simulink model "SMC_GRNN_Controller"  (R2019b)
settings: Solver=FixedStepAuto  StartTime=0.0  StopTime=60  FixedStep=1e-2  RelTol=1e-3
settings Model: Creator=Ivan Lopez  LastModifiedBy=Ivan Lopez

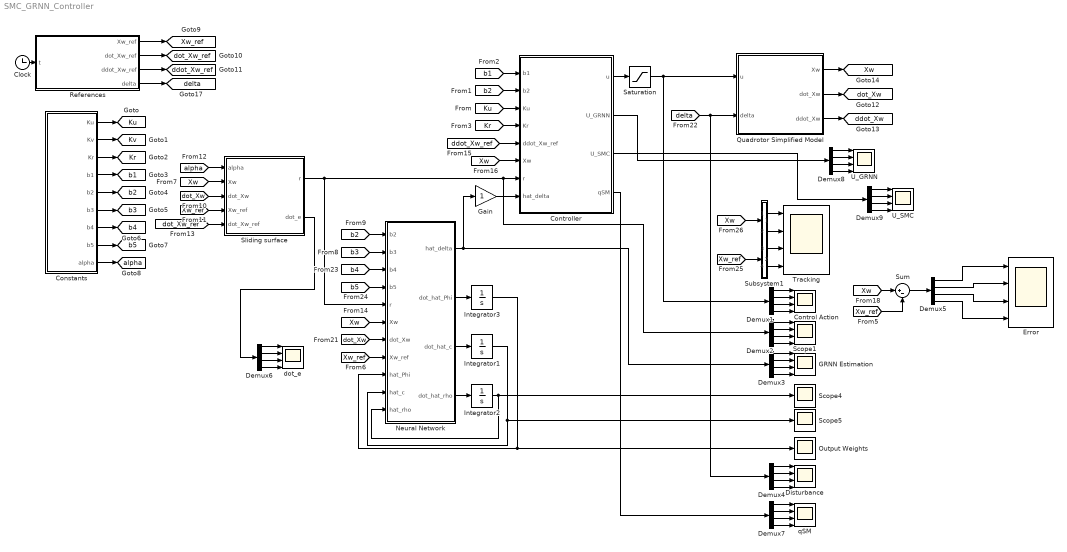
== system SMC_GRNN_Controller ==
  Clock : Clock
  Constants : MATLAB Function  TreatAsAtomicUnit=on
  Control Action : Scope  NumInputPorts=4
  Controller : MATLAB Function  TreatAsAtomicUnit=on
  Demux{1..9} (9 alike) : Demux
  Disturbance : Scope  NumInputPorts=4
  Error : Scope  NumInputPorts=4
  GRNN Estimation : Scope  NumInputPorts=4
  Gain : Gain
  Integrator1 : Integrator  InitialCondition=|
      | [0.6294
      |     0.8116
      |    -0.7460
      |     0.8268
      |     0.2647
      |    -0.8049
      |    -0.4430
      |     0.0938
      |     0.9150
      |     0.9298
      |    -0.6848
      |     0.9412
      |     0.9143
      |    -0.0292
      |     0.6006
      |    -0.7162
      |    -0.1565
      |     0.8315
      |     0.5844
      |     0.9190
      |     0.3115
      |    -0.9286
      |     0.6983
      |     0.8680
      |     0.3575
      |     0.5155
      |     0.4863
      |    -0.2155
      |     0.3110
      |    -0.6576
      |     0.4121
      |    -0.9363
      |    -0.4462
      |    -0.9077
      |    -0.8057
      |     0.6469
      |     0.3897
      |    -0.3658
      |     0.9004
      |    -0.9311
      |    -0.1225
      |    -0.2369
      |     0.5310
      |     0.5904
      |    -0.6263
      |    -0.0205
      |    -0.1088
      |     0.2926
      |     0.4187
      |     0.5094
      |    -0.4479
      |     0.3594
      |     0.3102
      |    -0.6748
      |    -0.7620
      |    -0.0033
      |     0.9195
      |    -0.3192
      |     0.1705
      |    -0.5524
      |     0.5025
      |    -0.4898
      |     0.0119
      |     0.3982
      |     0.7818
      |     0.9186
      |     0.0944
      |    -0.7228
      |    -0.7014
      |    -0.4850
      |     0.6814
      |    -0.4914
      |     0.6286
      |    -0.5130
      |     0.8585
      |    -0.3000
      |    -0.6068
      |    -0.4978
      |     0.2321
      |    -0.0534
      |    -0.2967
      |     0.6617
      |     0.1705
      |     0.0994
      |     0.8344
      |    -0.4283
      |     0.5144
      |     0.5075
      |    -0.2391
      |     0.1356
      |    -0.8483
      |    -0.8921
      |     0.0616
      |     0.5583
      |     0.8680
      |    -0.7402
      |     0.1376
      |    -0.0612
      |    -0.9762
      |    -0.3258
      |    -0.6756
      |     0.5886
      |    -0.3776
      |     0.0571
      |    -0.6687
      |     0.2040
      |    -0.4741
      |     0.3082
      |     0.3784
      |     0.4963
      |    -0.0989
      |    -0.8324
      |    -0.5420
      |     0.8267
      |    -0.6952
      |     0.6516
      |     0.0767
      |     0.9923
      |    -0.8436
      |    -0.1146
      |    -0.7867
      |     0.9238
      |    -0.9907
      |     0.5498
      |     0.6346
      |     0.7374
      |    -0.8311
      |    -0.2004
      |    -0.4803
      |     0.6001]'
  Integrator2 : Integrator  InitialCondition=ones(10,1)
  Integrator3 : Integrator  InitialCondition=|
      | [0.6628   -0.9690   -0.8946    0.3327;
      |     0.6067    0.9681    0.4757    0.0783;
      |    -0.8791   -0.6657   -0.4618    0.3962;
      |    -0.2015   -0.7876   -0.1543    0.3331;
      |     0.0538   -0.2552    0.0957   -0.6437;
      |    -0.1664   -0.6038    0.8855   -0.7440;
      |     0.3137   -0.0206   -0.1645    0.9982;
      |     0.2559   -0.3210    0.9661   -0.6578;
      |    -0.4160    0.9033   -0.3971   -0.9348;
      |    -0.1367    0.8407    0.4022    0.1224]
  Neural Network : MATLAB Function  TreatAsAtomicUnit=on
  Output Weights : Scope
  Quadrotor Simplified Model : Subsystem
  References : MATLAB Function  TreatAsAtomicUnit=on
  Saturation : Saturate  UpperLimit=1  LowerLimit=-1
  Scope1 : Scope  NumInputPorts=4
  Scope4 : Scope
  Scope5 : Scope
  Sliding surface : MATLAB Function  TreatAsAtomicUnit=on
  Subsystem1 : Subsystem
  Sum : Sum  Inputs=|+-
  Tracking : Scope  NumInputPorts=4
  U_GRNN : Scope  NumInputPorts=4
  U_SMC : Scope  NumInputPorts=4
  dot_e : Scope  NumInputPorts=4
  qSM : Scope  NumInputPorts=4
  tag scope: Kr=global, Ku=global, Kv=global, Xw=global, Xw_ref=global, alpha=global, b1=global, b2=global, b3=global, b4=global, b5=global, ddot_Xw=global, ddot_Xw_ref=global, delta=global, dot_Xw=global, dot_Xw_ref=global
  wires:
  References/3(ddot_Xw_ref) -> [ddot_Xw_ref]
  References/1(Xw_ref) -> [Xw_ref]
  References/2(dot_Xw_ref) -> [dot_Xw_ref]
  References/4(delta) -> [delta]
  Clock/1 -> References/1(t)
  Demux3/1 -> GRNN Estimation/1
  [Xw] -> Sliding surface/2(Xw)
  Demux3/3 -> GRNN Estimation/3
  [Ku] -> Controller/3(Ku)
  Neural Network/3(dot_hat_c) -> Integrator1/1
  Neural Network/1(hat_delta) -> Demux3/1, Gain/1
  [b5] -> Neural Network/4(b5)
  Integrator2/1 -> Scope4/1, Neural Network/11(hat_rho)
  Demux2/3 -> Scope1/3
  [b4] -> Neural Network/3(b4)
  Demux2/1 -> Scope1/1
  Constants/1(Ku) -> [Ku]
  [Xw] -> Controller/6(Xw)
  Demux2/4 -> Scope1/4
  Constants/2(Kv) -> [Kv]
  Constants/7(b4) -> [b4]
  [ddot_Xw_ref] -> Controller/5(ddot_Xw_ref)
  Constants/3(Kr) -> [Kr]
  Demux3/4 -> GRNN Estimation/4
  Demux3/2 -> GRNN Estimation/2
  Constants/8(b5) -> [b5]
  Sliding surface/1(r) -> Neural Network/5(r), Controller/7(r), Demux2/1
  [b2] -> Neural Network/1(b2)
  Demux1/4 -> Control Action/4
  [alpha] -> Sliding surface/1(alpha)
  Integrator1/1 -> Neural Network/10(hat_c), Scope5/1
  Constants/6(b3) -> [b3]
  [dot_Xw_ref] -> Sliding surface/5(dot_Xw_ref)
  [b3] -> Neural Network/2(b3)
  [Xw_ref] -> Neural Network/8(Xw_ref)
  [Kr] -> Controller/4(Kr)
  Constants/9(alpha) -> [alpha]
  [dot_Xw] -> Sliding surface/3(dot_Xw)
  Integrator3/1 -> Neural Network/9(hat_Phi), Output Weights/1
  Constants/5(b2) -> [b2]
  Demux1/3 -> Control Action/3
  [Xw] -> Neural Network/6(Xw)
  [b1] -> Controller/1(b1)
  Neural Network/2(dot_hat_Phi) -> Integrator3/1
  Neural Network/4(dot_hat_rho) -> Integrator2/1
  Constants/4(b1) -> [b1]
  Gain/1 -> Controller/8(hat_delta)
  Demux2/2 -> Scope1/2
  [Xw_ref] -> Sliding surface/4(Xw_ref)
  [b2] -> Controller/2(b2)
  [dot_Xw] -> Neural Network/7(dot_Xw)
  Quadrotor Simplified Model/3(ddot_Xw) -> [ddot_Xw]
  Quadrotor Simplified Model/2(dot_Xw) -> [dot_Xw]
  Quadrotor Simplified Model/1(Xw) -> [Xw]
  Subsystem1/1(Out1) -> Tracking/1
  Subsystem1/3(Out3) -> Tracking/3
  Subsystem1/2(Out2) -> Tracking/2
  [Xw] -> Subsystem1/1(In1)
  Subsystem1/4(Out4) -> Tracking/4
  [Xw_ref] -> Subsystem1/2(In2)
  Demux4/4 -> Disturbance/4
  Demux4/3 -> Disturbance/3
  Demux4/2 -> Disturbance/2
  Demux4/1 -> Disturbance/1
  [delta] -> Demux4/1, Quadrotor Simplified Model/2(delta)
  Controller/1(u) -> Saturation/1
  Saturation/1 -> Demux1/1, Quadrotor Simplified Model/1(u)
  Demux1/1 -> Control Action/1
  Demux1/2 -> Control Action/2
  [Xw] -> Sum/1
  [Xw_ref] -> Sum/2
  Sum/1 -> Demux5/1
  Demux5/2 -> Error/2
  Demux5/3 -> Error/3
  Demux5/1 -> Error/1
  Demux5/4 -> Error/4
  Demux6/3 -> dot_e/3
  Demux6/4 -> dot_e/4
  Demux6/1 -> dot_e/1
  Demux6/2 -> dot_e/2
  Sliding surface/2(dot_e) -> Demux6/1
  Demux7/2 -> qSM/2
  Demux7/3 -> qSM/3
  Controller/4(qSM) -> Demux7/1
  Demux7/1 -> qSM/1
  Demux7/4 -> qSM/4
  Demux8/2 -> U_GRNN/2
  Demux8/1 -> U_GRNN/1
  Demux8/3 -> U_GRNN/3
  Demux8/4 -> U_GRNN/4
  Controller/2(U_GRNN) -> Demux8/1
  Demux9/4 -> U_SMC/4
  Demux9/3 -> U_SMC/3
  Demux9/1 -> U_SMC/1
  Demux9/2 -> U_SMC/2
  Controller/3(U_SMC) -> Demux9/1

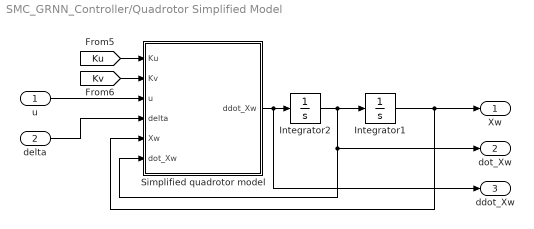
== system SMC_GRNN_Controller/Quadrotor Simplified Model ==
  u : Inport
  delta : Inport  Port=2
  Integrator1 : Integrator  InitialCondition=[0;0;0;0]  LimitOutput=on  UpperSaturationLimit=[inf;inf;inf;inf]  LowerSaturationLimit=[-inf;-inf;0;-inf]
  Integrator2 : Integrator  InitialCondition=[0;0;0;0]
  Simplified quadrotor model : MATLAB Function  TreatAsAtomicUnit=on
  Xw : Outport  VectorParamsAs1DForOutWhenUnconnected=off
  dot_Xw : Outport  Port=2  VectorParamsAs1DForOutWhenUnconnected=off
  ddot_Xw : Outport  Port=3  VectorParamsAs1DForOutWhenUnconnected=off
  wires:
  Simplified quadrotor model/1(ddot_Xw) -> ddot_Xw/1, Integrator2/1
  Integrator2/1 -> dot_Xw/1, Simplified quadrotor model/6(dot_Xw), Integrator1/1
  Integrator1/1 -> Xw/1, Simplified quadrotor model/5(Xw)
  [Ku] -> Simplified quadrotor model/1(Ku)
  delta/1 -> Simplified quadrotor model/4(delta)
  [Kv] -> Simplified quadrotor model/2(Kv)
  u/1 -> Simplified quadrotor model/3(u)

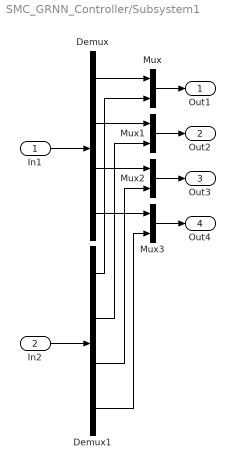
== system SMC_GRNN_Controller/Subsystem1 ==
  In1 : Inport
  In2 : Inport  Port=2
  Demux : Demux
  Demux1 : Demux
  Mux{,1..3} (4 alike) : Mux  Inputs=2
  Out1 : Outport  VectorParamsAs1DForOutWhenUnconnected=off
  Out2 : Outport  Port=2  VectorParamsAs1DForOutWhenUnconnected=off
  Out3 : Outport  Port=3  VectorParamsAs1DForOutWhenUnconnected=off
  Out4 : Outport  Port=4  VectorParamsAs1DForOutWhenUnconnected=off
  wires:
  Demux1/4 -> Mux3/2
  Demux1/1 -> Mux/2
  Demux/4 -> Mux3/1
  Demux1/3 -> Mux2/2
  Demux/2 -> Mux1/1
  Demux1/2 -> Mux1/2
  Demux/1 -> Mux/1
  Mux3/1 -> Out4/1
  Demux/3 -> Mux2/1
  Mux1/1 -> Out2/1
  In2/1 -> Demux1/1
  Mux/1 -> Out1/1
  In1/1 -> Demux/1
  Mux2/1 -> Out3/1

== matlab function SMC_GRNN_Controller/Controller ==
  data: b1 input; b2 input; Ku input; Kr input; ddot_Xw_ref input; u output; U_GRNN output; U_SMC output; Xw input; r input; hat_delta input; qSM output
function [u,U_GRNN,U_SMC,qSM] = fcn(b1,b2,Ku,Kr,ddot_Xw_ref,Xw,r,hat_delta)

psi = Xw(4);

R = [cos(psi)  sin(psi)  0  0;
     sin(psi)  -cos(psi)  0  0;
     0          0         1  0;
     0          0         0  1];

U = (R*Ku)\(ddot_Xw_ref - b1*tanh(b2*r) - hat_delta - Kr*sign(r));
U_GRNN = (R*Ku)\(- hat_delta);
U_SMC = (R*Ku)\(ddot_Xw_ref - b1*tanh(b2*r) - Kr*sign(r));
qSM = b1*tanh(b2*r);
% U = (R*Ku)\(-b1*r - 0*hat_delta);
% U = b1*tanh(b2*r) - Kr*sign(r);
u = [U(1);U(2);U(3);U(4)];

== matlab function SMC_GRNN_Controller/Quadrotor Simplified Model/Simplified quadrotor model ==
  data: Ku input; Kv input; u input; delta input; Xw input; dot_Xw input; ddot_Xw output
function ddot_Xw = fcn(Ku,Kv,u,delta,Xw,dot_Xw)

psi = Xw(4);

R = [cos(psi)  sin(psi)  0  0;
     sin(psi)  -cos(psi)  0  0;
     0          0         1  0;
     0          0         0  1];

ddot_Xw = R*Ku*u - Kv*dot_Xw + delta;

== matlab function SMC_GRNN_Controller/Neural Network ==
  settings: updateMethod=DISCRETE
  data: b2 input; b3 input; b4 input; b5 input; r input; Xw input; dot_Xw input; Xw_ref input; hat_Phi input; hat_delta output; dot_hat_Phi output; hat_c input; dot_hat_c output; hat_rho input; dot_hat_rho output
function [hat_delta,dot_hat_Phi,dot_hat_c,dot_hat_rho] = fcn(b2,b3,b4,b5,r,Xw,dot_Xw,Xw_ref,hat_Phi,hat_c,hat_rho)

e = Xw - Xw_ref;
bar_r = [1;e;r;dot_Xw]; % Extended Input Vector

% Neural network constants
m   = 10; % Neurons Quantity
E   = numel(bar_r); % Input Quantity of the Neural Network
n   = 4; % Output Quantity of the Neural Network
% rho = ones(m,1); % Variance Vector

% -1 + (1-(-1)).*rand(m,n); % Random values from -1 to 1 to initialize the integrator

hat_c_m = zeros(E,m);
cont = 0;
for i = 1:m
    for j = 1:E
        hat_c_m(j,i) = hat_c(cont*E+j); % Mean Value Matrix
    end
    cont = cont + 1;
end

% Activation Function
H = zeros(m,1);
for i = 1:m
    sum1 = 0;
    for j = 1:m
        sum1 = sum1 + exp(norm(bar_r-hat_c_m(:,j))/(2*hat_rho(j)));
    end
    H(i,1) = exp(norm(bar_r-hat_c_m(:,i))/(2*hat_rho(i)))/sum1; % Gaussian with mean z and variance rho
end

% Adaptation Law for output weights
dot_hat_Phi = zeros(m,n);
for i = 1:n
    dot_hat_Phi(:,i) = b3*H*tanh(b2*r(i));
end

% Adaptation of the mean vector
% Sumatoria del denominador de la derivada parcial de Hi con respecto a ci
sum2 = 0;
for i = 1:m
    sum2 = sum2 + exp(norm(bar_r - hat_c_m(:,i))/(2*hat_rho(i))); % Sumation
end
% Derivada parcial del Hi con respecto de cij
dot_Hc = zeros(m,m,E);
for i = 1:m
    for j = 1:m
        for k = 1:E
            if j==i
                num1 = exp(norm(bar_r - hat_c_m(:,j))/(2*hat_rho(j)));
                num2 = -((bar_r(k) - hat_c_m(k,j))/(2*hat_rho(j)*norm(bar_r - hat_c_m(:,j)))); % NOTA hat_c_m es de E X m
                num3 = exp(norm(bar_r - hat_c_m(:,j))/(hat_rho(j)));
                dot_Hc(i,j,k) = (num1*num2*sum2 - num3*num2)/sum2^2;
            else
                num4 = -exp((norm(bar_r - hat_c_m(:,i)))/(2*hat_rho(i)));
                num5 = -((bar_r(k) - hat_c_m(k,j))/(2*hat_rho(j)*norm(bar_r - hat_c_m(:,j)))); % NOTA hat_c_m es de E X m
                num6 = exp(norm(bar_r - hat_c_m(:,j))/(hat_rho(j)));
                dot_Hc(i,j,k) = (num4*num5*num6)/sum2^2;
            end
        end
    end
end
DHc = reshape(permute(dot_Hc,[1 3 2]),m,(m*E)); % Construccion de la matriz
% Adaptation Law for mean vector
sumation_c = zeros(E*m,1);
for i = 1:4
    sumation_c = sumation_c + tanh(b2*r(i))*DHc'*hat_Phi(:,i);
end

dot_hat_c = b4*sumation_c;

% Adaptation of the variance vector
DHrho = zeros(m,1);
for i = 1:m
    num7 = -norm(bar_r - hat_c_m(:,i))/(2*hat_rho(i)^2);
    num8 = exp((norm(bar_r - hat_c_m(:,i)))/(2*hat_rho(i)));
    DHrho(i,1) = (sum2*num7*num8 - num8^2*num7)/sum2^2;
end
% Adaptation Law for variance vector
sumation_rho = zeros(m,1);
for i = 1:4
    sumation_rho = sumation_rho + tanh(b2*r(i))*DHrho'*hat_Phi(:,i);
end

dot_hat_rho = b5*sumation_rho;

% Neural network
hat_delta = hat_Phi'*H;

== matlab function SMC_GRNN_Controller/References ==
  data: Xw_ref output; dot_Xw_ref output; ddot_Xw_ref output; t input; delta output
function [Xw_ref,dot_Xw_ref,ddot_Xw_ref,delta]= fn(t)

xamp = 0.5;
yamp = 1.0;
zamp = 0.4;
xfr = 2*pi/4;
yfr = 2*pi/8;
zfr = 2*pi/4;

x_ref   = xamp*sin(xfr*t);
y_ref   = yamp*cos(yfr*t);
z_ref   = 1.0 + zamp*sin(zfr*t);
psi_ref = 0.0;

dot_x_ref   = xamp*xfr*cos(xfr*t);
dot_y_ref   = -yamp*yfr*sin(yfr*t);
dot_z_ref   = zamp*zfr*cos(zfr*t);
dot_psi_ref = 0.0;

ddot_x_ref   = -xamp*xfr^2*sin(xfr*t);
ddot_y_ref   = -yamp*yfr^2*cos(yfr*t);
ddot_z_ref   = -zamp*zfr^2*sin(zfr*t);
ddot_psi_ref = 0.0;

delta = [0.0
         0.0
         0.0
         0.0];

if ((t>= 40))
    delta = [1*sin((2*pi*t)/4)
             1*cos((2*pi*t)/8)
             1*sin((2*pi*t)/4)
             1*sin((2*pi*t)/4)];
end
Xw_ref      = [x_ref;y_ref;z_ref;psi_ref];
dot_Xw_ref  = [dot_x_ref;dot_y_ref;dot_z_ref;dot_psi_ref];
ddot_Xw_ref = [ddot_x_ref;ddot_y_ref;ddot_z_ref;ddot_psi_ref];

== matlab function SMC_GRNN_Controller/Constants ==
  data: Ku output; Kv output; Kr output; b1 output; b2 output; b3 output; b4 output; b5 output; alpha output
function [Ku,Kv,Kr,b1,b2,b3,b4,b5,alpha] = fcn()

% Model parameters
Ku = diag([4.72;6.23;2.65;2.38]);
Kv = diag([0.28;0.53;2.58;1.52]);

% Controller gains
Kr = 0.001*diag([1;1;1;1]);

% Saturation function coeff
b1 = 0.75;
b2 = 30;
% Neural Network Constants
b3 = 1*26; % Neural Network gain
b4 = 0.8; % Mean vector adaptation gain
b5 = 0.8; % Variance vector adaptation gain

% Sliding surface gains
alpha = 0.15*diag([1.5;1.5;4.8;1.5]);

== matlab function SMC_GRNN_Controller/Sliding surface ==
  data: alpha input; Xw input; r output; dot_Xw input; Xw_ref input; dot_Xw_ref input; dot_e output
function [r,dot_e]  = fcn(alpha,Xw,dot_Xw,Xw_ref,dot_Xw_ref)

e      = Xw - Xw_ref;
dot_e  = dot_Xw - dot_Xw_ref;
r      = dot_e + alpha*e;
